simulink model "APFC_FullModel_v22_NoALPF"  (R2025b)
settings: Solver=ode23t  StartTime=0.0  StopTime=50  MaxStep=2e-4  RelTol=1e-3
undefined symbols (not defined in the file): a_dq, ALPF_fs, b_dq, C_B1, C_B2, C_B3, DiscIntNeverNeededParam, dspblkCoreblockFVToolHelper, FLC_deadband_kVAR, gcbh, L_B1, L_B2, L_B3, omega, p, Q_reactor, Rc, tau_Qload, X1
libraries: ee_lib x63, fl_lib x59, nesl_utility x43, dspswit3 x9, eeTransforms x2, fuzblock x1, eeSinusoidalMeasurementV2 x1
(part 1 of 4)
settings Model: Creator=User  LastModifiedBy=User
settings SolverCC: MaxConsecutiveMinStep=1000

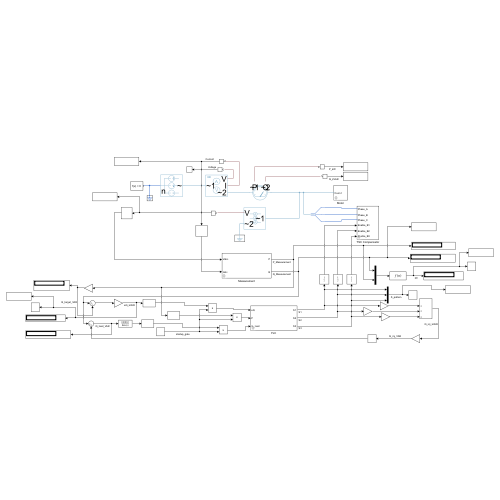
[thumbnail: Simulink's stored preview of the top-level diagram]
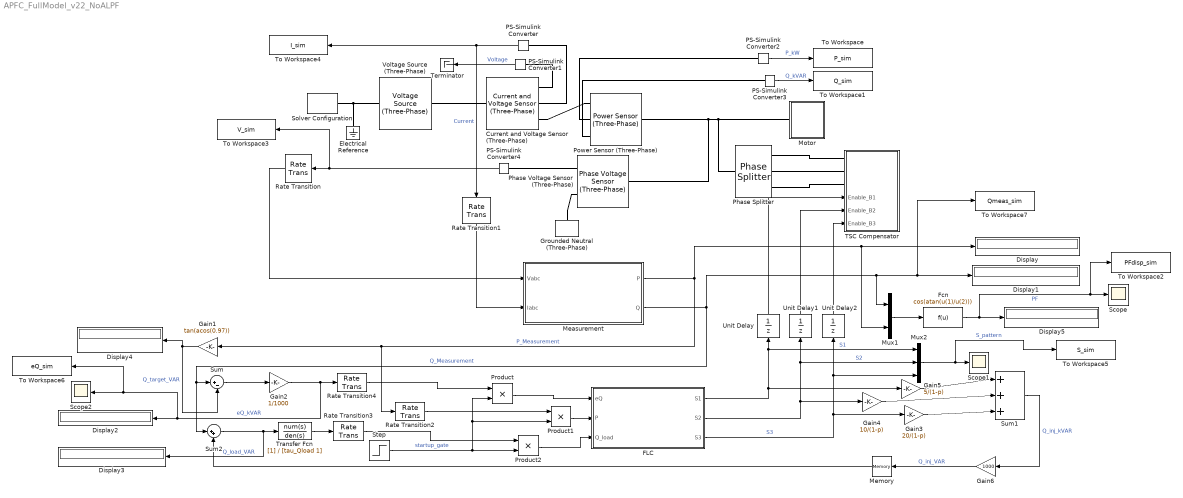
== system APFC_FullModel_v22_NoALPF ==
  Current and Voltage Sensor (Three-Phase) : ee_lib/Sensors & Transducers/Current and Voltage Sensor (Three-Phase)  vMeasurementType=ee.enum.vmeasurement.ll  outputUnit=ee.enum.unit.si  SRated=100e6 A*V  VRated=24e3 V  I_specify=off  I_priority=None  I=[0, 0, 0] A  I_nominal_specify=off  I_nominal_value=1  I_nominal_unit=A  V_specify=off  V_priority=None  V=[0, 0, 0] V  V_nominal_specify=off  V_nominal_value=1  V_nominal_unit=V
      settings: InternalSimscapePortConfiguration="{\"Bottom\":[],\"Left\":[{\"id\":\"N1\",\"label\":\"~1\",\"type\":\"foundation.electrical.three_phase\"}],\"Right\":[{\"id\":\"V_output\",\"label\":\"V\",\"type\":\"output\"},{\"id\":\"I_output\",\"label\":\"I\",\"type\":\"output\"},{\"id\":\"N2\",\"label\":\"~2\",\"type\":\"foundation.electrical.three_phase\"}],\"Top\":[]}"
  Display{,1..5} (6 alike) : Display
  Electrical Reference : fl_lib/Electrical/Electrical Elements/Electrical Reference
  FLC : Subsystem  mask(Fuzzy Logic Controller){}
      mask help: Reads eQ, P, Q_load; fuzzy inference plus deterministic PF-floor; outputs bank commands S1/S2/S3. Parameters sourced from APFC_Parameters.m.
  Fcn : Fcn  Expr=cos(atan(u(1)/u(2)))
  Gain1 : Gain  Gain=tan(acos(0.97))
  Gain2 : Gain  Gain=1/1000
  Gain3 : Gain  Gain=20/(1-p)
  Gain4 : Gain  Gain=10/(1-p)
  Gain5 : Gain  Gain=5/(1-p)
  Gain6 : Gain  Gain=1000
  Grounded Neutral (Three-Phase) : ee_lib/Connectors & References/Grounded Neutral (Three-Phase)
  Measurement : Subsystem  mask(Measurement){}
      mask help: Vabc, Iabc → P, Q. Native Sinusoidal Measurement (PLL, Three-Phase) + Park Transform; alignment-agnostic instantaneous-power computation. Shared PLL angle for both transforms.
  Memory : Memory
  Motor : Subsystem  mask(APFC Motor){n_rpm=1485}
      mask prompts: n_rpm "Rotor speed (rpm)"
      mask help: 30 kW squirrel-cage induction machine with core-loss shunt (Rc), grounded neutral, and speed-imposed mechanical drive. Electrical parameters from APFC_Parameters.m. Rotor speed set via n_rpm.
  Mux1 : Mux  Inputs=2
  Mux2 : Mux  Inputs=3
  PS-Simulink Converter{,1..4} (5 alike) : nesl_utility/PS-Simulink Converter  PhysicalDomain=network_engine_domain  SubClassName=ps_output  LeftPortType=input  RightPortType=output  PseudoPeriodic=off  Frequencies=[]  VectorFormat=inherit  Unit=inherit  AffineConversion=off
  Phase Splitter : ee_lib/Connectors & References/Phase Splitter
  Phase Voltage Sensor (Three-Phase) : ee_lib/Sensors & Transducers/Phase Voltage Sensor (Three-Phase)
  Power Sensor (Three-Phase) : ee_lib/Sensors & Transducers/Power Sensor (Three-Phase)  load_type=ee.enum.passive.type_balanced.balanced  f0=50 Hz
      settings: InternalSimscapePortConfiguration="{\"Bottom\":[],\"Left\":[{\"id\":\"N1\",\"label\":\"~1\",\"type\":\"foundation.electrical.three_phase\"}],\"Right\":[{\"id\":\"N2\",\"label\":\"~2\",\"type\":\"foundation.electrical.three_phase\"}],\"Top\":[{\"id\":\"Pm\",\"label\":\"P\",\"type\":\"output\"},{\"id\":\"Qm\",\"label\":\"Q\",\"type\":\"output\"}]}"
  Product : Product
  Product1 : Product
  Product2 : Product
  Rate Transition : RateTransition  Deterministic=off  OutPortSampleTime=1/12500
  Rate Transition1 : RateTransition  Deterministic=off  OutPortSampleTime=1/12500
  Rate Transition2 : RateTransition  OutPortSampleTime=0.5
  Rate Transition3 : RateTransition  OutPortSampleTime=0.5
  Rate Transition4 : RateTransition  OutPortSampleTime=0.5
  Scope : Scope
      settings: ActiveDisplayYMinimum=-0.12495061956957584  ActiveDisplayYMaximum=1.1249945132855084
  Scope1 : Scope
      settings: ActiveDisplayYMinimum=-0.12499999999999997  ActiveDisplayYMaximum=1.125  DataLoggingVariableName=ScopeData3
  Scope2 : Scope
      settings: ActiveDisplayYMinimum=-28.043898600792488  ActiveDisplayYMaximum=214.93630943141093  DataLoggingVariableName=ScopeData4
  Solver Configuration : nesl_utility/Solver Configuration  PhysicalDomain=network_engine_domain  SubClassName=solver  LeftPortType=input  RightPortType=generic  Tones=[]  Harmonics=[]  SimulateNoise=off  Profile=off  UseLocalSampling=off  EnableSwitchedLinearOptims=on  FrequencyDomain=off  UseCCode=off  RelTol=0.001  AbsTol=0.001  MinStep=1e-09  ToWorkspace=off  RevertToSquareIcSolve=off  NumHomotopyIterations=100  PhasorMode=off  PhasorModeNumHarmonics=1  ConsistencySolver=NEWTON_XTOL_AFTER_FTOL  IndexReductionMethod=DerivativeReplacement  DoDC=off  ResidualTolerance=1e-09  ConsistencyTolSource=GLOBAL  ConsistencyAbsTol=0.001  ConsistencyRelTol=0.001  ConsistencyTolFactor=0.01  UseLocalSolver=off  LocalSolverChoice=NE_BACKWARD_EULER_ADVANCER  ResolveIndetEquations=on  FunctionEvalNumThread=1  LocalSolverSampleTime=0.001  DoFixedCost=off  MaxNonlinIter=3  MaxModeIter=2  ComputeImpulses=off  ImpulseIterations=2  LinearAlgebra=auto  LinearAlgebraNumThread=0  EquationFormulation=NE_TIME_EF  DelaysMemoryBudget=1024  AutomaticFiltering=on  FilteringTimeConstant=0.001  PartitionStorageMethod=AS_NEEDED  PartitionMemoryBudget=1024  PartitionMethod=ROBUST  MultibodyUseLocalSolver=off  MultibodyLocalSolverChoice=ODE1  MultibodyLocalSolverSampleTime=0.001
  Step : Step  Time=25  SampleTime=0.5
  Sum : Sum  Inputs=|+-
  Sum1 : Sum  Inputs=|+++
  Sum2 : Sum  Inputs=|++
  TSC Compensator : Subsystem  mask(TSC Compensator){}
      mask help: Three-phase, delta-connected thyristor-switched capacitor compensator. Three binary-weighted banks: Bank_1 = 5 kVAR, Bank_2 = 10 kVAR, Bank_3 = 20 kVAR (nominal capacitor rating) at 415 V / 50 Hz, 6 % detuned, delivering 5.32 / 10.64 / 21.28 kVAR to the network. Each bank is enabled via Enable_B1/B2/B3 with ZCD-latched transient-free switching. Capacitance and inductance are set inside each bank's Delta_Limb masks — not at this level. Ports: physical Phase_A/B/C; signal Enable_B1/B2/B3.
      settings: PortSchema="{\"entries\":[{\"content\":{\"sides\":[{\"content\":{\"connectorIds\":[\"LConn1\",\"LConn2\",\"LConn3\",\"In1\",\"In2\",\"In3\"]},\"type\":\"ConnectorPlacement.EquallySpacedRectSide\",\"uuid\":\"f449d328-b061-4fce-b527-12937b4bf208\"},{\"content\":{\"side\":\"RIGHT\"},\"type\":\"ConnectorPlacement.EquallySpacedRectSide\",\"uuid\":\"515dffab-51bf-4c86-87e0-d575b9a1f73c\"},{\"content\":{\"side\":\"TOP\"},\"type\":\"ConnectorPlacement.EquallySpacedRectSide\",\"uuid\":\"b4eb947e-b77f-4dcc-ae55-0412ff2259e4\"}]},\"type\":\"ConnectorPlacement.EquallySpacedConnector\",\"uuid\":\"1bf47cce-5631-4349-8217-69cf3260ee1b\"}],\"packageUris\":[\"http://schema.mathworks.com/mf0/Connector/R2020b\"],\"version\":\"1.0\"}"
  Terminator : Terminator
  To Workspace : ToWorkspace  VariableName=P_sim  SampleTime=-1
  To Workspace1 : ToWorkspace  VariableName=Q_sim  SampleTime=-1
  To Workspace2 : ToWorkspace  VariableName=PFdisp_sim  SaveFormat=Timeseries  SampleTime=-1
  To Workspace3 : ToWorkspace  VariableName=V_sim  SampleTime=-1
  To Workspace4 : ToWorkspace  VariableName=I_sim  SampleTime=-1
  To Workspace5 : ToWorkspace  VariableName=S_sim  SaveFormat=Timeseries  SampleTime=-1
  To Workspace6 : ToWorkspace  VariableName=eQ_sim  SaveFormat=Timeseries  SampleTime=-1
  To Workspace7 : ToWorkspace  VariableName=Qmeas_sim  SaveFormat=Timeseries  SampleTime=-1
  Transfer Fcn : TransferFcn  Denominator=[tau_Qload 1]
  Unit Delay : UnitDelay  SampleTime=0.5  HasFrameUpgradeWarning=on
  Unit Delay1 : UnitDelay  SampleTime=0.5  HasFrameUpgradeWarning=on
  Unit Delay2 : UnitDelay  SampleTime=0.5  HasFrameUpgradeWarning=on
  Voltage Source (Three-Phase) : ee_lib/Sources/Voltage Source (Three-Phase)  vline_rms=415 V  shift=0 deg  freq=50 Hz  impedance_option=2  SShortCircuit=1e6 A*V  XR=15  R=0.001 Ohm  L=3.97e-4 H  harmonic_option=1  harmonic_orders=H_orders  harmonic_ratios=H_ratios  G_parasitic=0 1/Ohm  I_specify=off  I_priority=None  I=[0, 0, 0] A  I_nominal_specify=off  I_nominal_value=1  I_nominal_unit=A
  wires:
  PS-Simulink Converter/1 -> To Workspace4/1, Rate Transition1/1  "Current"
  PS-Simulink Converter3/1 -> To Workspace1/1  "Q_kVAR"
  PS-Simulink Converter2/1 -> To Workspace/1  "P_kW"
  PS-Simulink Converter4/1 -> To Workspace3/1, Rate Transition/1
  Rate Transition/1 -> Measurement/1(Vabc)
  Rate Transition1/1 -> Measurement/2(Iabc)
  Measurement/2(Q) -> Sum2/1, Sum/1, Mux1/1, To Workspace7/1, Display1/1  "Q_Measurement"
  Measurement/1(P) -> Rate Transition2/1, Gain1/1, Mux1/2, Display/1  "P_Measurement"
  Gain1/1 -> Sum/2, Display4/1  "Q_target_VAR"
  Sum/1 -> Gain2/1
  Sum1/1 -> Gain6/1  "Q_inj_kVAR"
  Gain6/1 -> Memory/1  "Q_inj_VAR"
  Memory/1 -> Sum2/2
  Gain2/1 -> To Workspace6/1, Scope2/1, Display2/1, Rate Transition4/1  "eQ_kVAR"
  Sum2/1 -> Display3/1, Transfer Fcn/1  "Q_load_VAR"
  Product/1 -> FLC/1(eQ)
  Product1/1 -> FLC/2(P)
  Product2/1 -> FLC/3(Q_load)
  Step/1 -> Product1/2, Product/2, Product2/2  "startup_gate"
  Rate Transition3/1 -> Product2/1
  Rate Transition2/1 -> Product1/1
  Rate Transition4/1 -> Product/1
  FLC/3(S3) -> Unit Delay2/1, Mux2/3, Gain3/1  "S3"
  FLC/2(S2) -> Unit Delay1/1, Mux2/2, Gain4/1  "S2"
  FLC/1(S1) -> Unit Delay/1, Mux2/1, Gain5/1  "S1"
  Gain3/1 -> Sum1/3
  Gain4/1 -> Sum1/2
  Gain5/1 -> Sum1/1
  Unit Delay2/1 -> TSC Compensator/3(Enable_B3)
  Unit Delay1/1 -> TSC Compensator/2(Enable_B2)
  Unit Delay/1 -> TSC Compensator/1(Enable_B1)
  Mux1/1 -> Fcn/1
  Fcn/1 -> To Workspace2/1, Scope/1, Display5/1  "PF"
  Mux2/1 -> To Workspace5/1, Scope1/1  "S_pattern"
  Transfer Fcn/1 -> Rate Transition3/1
  PS-Simulink Converter1/1 -> Terminator/1  "Voltage"
  connections:
  Current and Voltage Sensor (Three-Phase)/RConn3 -- Power Sensor (Three-Phase)/LConn1
  Electrical Reference/LConn1 -- Voltage Source (Three-Phase)/LConn1 -- Solver Configuration/RConn1
  PS-Simulink Converter1/LConn1 -- Current and Voltage Sensor (Three-Phase)/RConn1
  PS-Simulink Converter/LConn1 -- Current and Voltage Sensor (Three-Phase)/RConn2
  Voltage Source (Three-Phase)/RConn1 -- Current and Voltage Sensor (Three-Phase)/LConn1
  Phase Splitter/RConn2 -- TSC Compensator/LConn2
  Phase Splitter/RConn3 -- TSC Compensator/LConn3
  Phase Splitter/RConn1 -- TSC Compensator/LConn1
  Power Sensor (Three-Phase)/RConn1 -- Phase Voltage Sensor (Three-Phase)/LConn1 -- Phase Splitter/LConn1 -- Motor/LConn1
  Grounded Neutral (Three-Phase)/LConn1 -- Phase Voltage Sensor (Three-Phase)/RConn2
  Phase Voltage Sensor (Three-Phase)/RConn1 -- PS-Simulink Converter4/LConn1
  PS-Simulink Converter3/LConn1 -- Power Sensor (Three-Phase)/LConn3
  PS-Simulink Converter2/LConn1 -- Power Sensor (Three-Phase)/LConn2

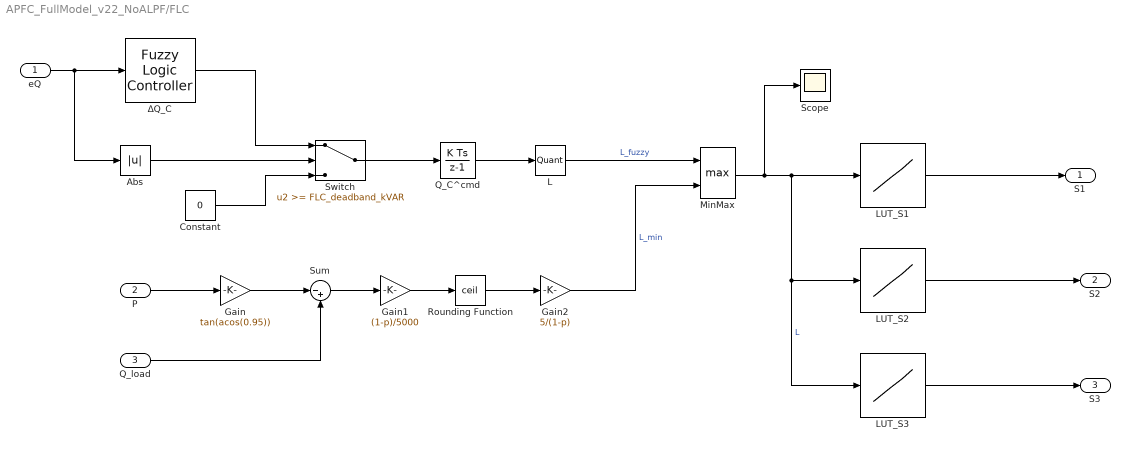
== system APFC_FullModel_v22_NoALPF/FLC ==
  eQ : Inport
  P : Inport  Port=2
  Q_load : Inport  Port=3
  Abs : Abs  SaturateOnIntegerOverflow=off
  Constant : Constant  Value=0
  Gain : Gain  Gain=tan(acos(0.95))
  Gain1 : Gain  Gain=(1-p)/5000
  Gain2 : Gain  Gain=5/(1-p)
  L : Quantizer  QuantizationInterval=5/(1-p)
  LUT_S1 : Lookup_n-D  NumberOfTableDimensions=1  BreakpointsForDimension1=(0:7)*(5/(1-p))  Table=[0 1 0 1 0 1 0 1]  InterpMethod=Flat  InternalRulePriority=Speed  RndMeth=Simplest
  LUT_S2 : Lookup_n-D  NumberOfTableDimensions=1  BreakpointsForDimension1=(0:7)*(5/(1-p))  Table=[0 0 1 1 0 0 1 1]  InterpMethod=Flat  InternalRulePriority=Speed  RndMeth=Simplest
  LUT_S3 : Lookup_n-D  NumberOfTableDimensions=1  BreakpointsForDimension1=(0:7)*(5/(1-p))  Table=[0 0 0 0 1 1 1 1]  InterpMethod=Flat  InternalRulePriority=Speed  RndMeth=Simplest
  MinMax : MinMax  Function=max  Inputs=2
  Q_C^cmd : DiscreteIntegrator  gainval=0.2  SampleTime=0.5  LimitOutput=on  UpperSaturationLimit=35/(1-p)  LowerSaturationLimit=0  ICPrevOutput=DiscIntNeverNeededParam  ICPrevScaledInput=DiscIntNeverNeededParam
  Rounding Function : Rounding  Operator=ceil
  Scope : Scope
      settings: ActiveDisplayYMinimum=5.9574468085106389  ActiveDisplayYMaximum=25.957446808510639  DataLoggingVariableName=ScopeData2
  Sum : Sum  Inputs=|-+
  Switch : Switch  Threshold=FLC_deadband_kVAR  SaturateOnIntegerOverflow=off  InputSameDT=off
  ΔQ_C : fuzblock/Fuzzy Logic  Controller  FIS=fis  OutputSampleNumber=101  DataType=double  UseLookupTable=off  NumBreakpoints=10  FuzzifiedInputs=off  RuleFiringStrengths=off  RuleOutputs=off  AggregatedOutputs=off  SimulateUsing=Interpreted execution  OutOfRangeInputValueMessage=warning  NoRuleFiredMessage=warning  EmptyOutputFuzzySetMessage=warning
  S1 : Outport
  S2 : Outport  Port=2
  S3 : Outport  Port=3
  wires:
  Q_C^cmd/1 -> L/1
  LUT_S3/1 -> S3/1
  eQ/1 -> Abs/1, ΔQ_C/1
  LUT_S1/1 -> S1/1
  LUT_S2/1 -> S2/1
  Switch/1 -> Q_C^cmd/1
  ΔQ_C/1 -> Switch/1
  Abs/1 -> Switch/2
  Constant/1 -> Switch/3
  P/1 -> Gain/1
  Gain/1 -> Sum/1
  Q_load/1 -> Sum/2
  Sum/1 -> Gain1/1
  Gain1/1 -> Rounding Function/1
  Rounding Function/1 -> Gain2/1
  MinMax/1 -> Scope/1, LUT_S3/1, LUT_S2/1, LUT_S1/1  "L"
  L/1 -> MinMax/1  "L_fuzzy"
  Gain2/1 -> MinMax/2  "L_min"

== system APFC_FullModel_v22_NoALPF/Measurement ==
  Vabc : Inport
  Iabc : Inport  Port=2
  Demux : Demux  Outputs=3
  Demux1 : Demux  Outputs=3
  Discrete Transfer Fcn : DiscreteTransferFcn  LoadFcn=dspblkCoreblockFVToolHelper(gcbh,'load');  Numerator=[b_dq]  Denominator=[1 -a_dq]
      settings: CopyFcn=dspblkCoreblockFVToolHelper(gcbh,'copy');  DeleteFcn=dspblkCoreblockFVToolHelper(gcbh,'close');  ModelCloseFcn=dspblkCoreblockFVToolHelper(gcbh,'close');  PreSaveFcn=dspblkCoreblockFVToolHelper(gcbh,'presave');  PostSaveFcn=dspblkCoreblockFVToolHelper(gcbh,'postsave');  CloseFcn=dspblkCoreblockFVToolHelper(gcbh,'close');
  Discrete Transfer Fcn1 : DiscreteTransferFcn  LoadFcn=dspblkCoreblockFVToolHelper(gcbh,'load');  Numerator=[b_dq]  Denominator=[1 -a_dq]
      settings: CopyFcn=dspblkCoreblockFVToolHelper(gcbh,'copy');  DeleteFcn=dspblkCoreblockFVToolHelper(gcbh,'close');  ModelCloseFcn=dspblkCoreblockFVToolHelper(gcbh,'close');  PreSaveFcn=dspblkCoreblockFVToolHelper(gcbh,'presave');  PostSaveFcn=dspblkCoreblockFVToolHelper(gcbh,'postsave');  CloseFcn=dspblkCoreblockFVToolHelper(gcbh,'close');
  Mux2 : Mux
  P-Fcn : Fcn  Expr=1.5*(u(1)*u(3)+u(2)*u(4))
  Park Transform : eeTransforms/Park Transform  AxisAlignment=D-axis  PowerInvariant=off
      settings: LibrarySourceBlock=|
      | ee_sl_lib/Mathematical
      | Transforms/Park Transform
  Park Transform1 : eeTransforms/Park Transform  AxisAlignment=D-axis  PowerInvariant=off
      settings: LibrarySourceBlock=|
      | ee_sl_lib/Mathematical
      | Transforms/Park Transform
  Q-Fcn : Fcn  Expr=1.5*(u(2)*u(3)-u(1)*u(4))
  Scope : Scope
      settings: ActiveDisplayYMinimum=-1  ActiveDisplayYMaximum=1
  "Sinusoidal Measurement (PLL, Three-Phase)" : eeSinusoidalMeasurementV2/Sinusoidal Measurement (PLL, Three-Phase)  InputFilter=on  InputNormalization=off  Kp_LF=1  Ki_LF=10  F0=50  Theta0=0  Ts=1/ALPF_fs
      settings: LibrarySourceBlock=|
      | ee_sl_lib/Measurements/Sinusoidal Measurement
      | (PLL, Three-Phase)
  Terminator{,1..3} (4 alike) : Terminator
  P : Outport
  Q : Outport  Port=2
  wires:
  Park Transform/1 -> Demux/1
  Park Transform1/1 -> Demux1/1
  Demux/1 -> Mux2/1  "Vd"
  P-Fcn/1 -> Discrete Transfer Fcn/1
  Demux/3 -> Terminator2/1
  "Sinusoidal Measurement (PLL, Three-Phase)"/2 -> Scope/1, Park Transform1/2, Park Transform/2
  Demux/2 -> Mux2/2  "Vq"
  "Sinusoidal Measurement (PLL, Three-Phase)"/3 -> Terminator1/1
  Vabc/1 -> Park Transform/1, "Sinusoidal Measurement (PLL, Three-Phase)"/1
  Demux1/3 -> Terminator3/1
  "Sinusoidal Measurement (PLL, Three-Phase)"/1 -> Terminator/1
  Mux2/1 -> Q-Fcn/1, P-Fcn/1
  Iabc/1 -> Park Transform1/1
  Q-Fcn/1 -> Discrete Transfer Fcn1/1
  Discrete Transfer Fcn/1 -> P/1
  Demux1/1 -> Mux2/3  "Id"
  Demux1/2 -> Mux2/4  "Iq"
  Discrete Transfer Fcn1/1 -> Q/1

== system APFC_FullModel_v22_NoALPF/Motor ==
  Grounded Neutral (Three-Phase) : ee_lib/Connectors & References/Grounded Neutral (Three-Phase)
  Ideal Angular Velocity Source : fl_lib/Mechanical/Mechanical Sources/Ideal Angular Velocity Source
  Induction Machine Squirrel Cage : ee_lib/Electromechanical/Asynchronous/Induction Machine Squirrel Cage  port_option=ee.enum.threePhasePort.composite  SRated=SIn_3ph A*V  VRated=415 V  FRated=50 Hz  nPolePairs=2  param_unit=ee.enum.unit.si  squirrel_cage=ee.enum.squirrelcage.Single  zero_sequence=ee.enum.park.zerosequence.exclude  initialization_option=ee.enum.asm.initialization.fluxvariables  Rs=R1 Ohm  Xls=X1 Ohm  pu_Rs=0.0258  pu_Lls=0.0413  Rrd=R2 Ohm  Xlrd=X2 Ohm  pu_Rrd=0.0145  pu_Llrd=0.0424  Rrd1=0.28 Ohm  Xlrd1=0.82 Ohm  Rrd2=0.28 Ohm  Xlrd2=0.82 Ohm  pu_Rrd1=0.0290  pu_Llrd1=0.0848  pu_Rrd2=0.0290  pu_Llrd2=0.0848  Xm=XM Ohm  pu_Lm=1.7562  X0=X1 Ohm  pu_L0=0.0413  saturation_option=ee.enum.saturation.exclude  saturation_i=[0, 4, 9, 18, 25, 34, 50, 68, 95, 120] A  saturation_v=[0, 88, 154, 198, 220, 242, 264, 286, 308, 327] V  pu_saturation_i=[0, .176, .396, .792, 1.1, 1.496, 2.2, 2.992, 4.18, 5.28]  pu_saturation_v=[0, .4, .7, .9, 1, 1.1, 1.2, 1.3, 1.4, 1.4864]  connection_option=ee.enum.Connection.delta  angular_position_specify=off  angular_position_priority=None  angular_position=0 deg  angular_position_nominal_specify=off  angular_position_nominal_value=1  angular_position_nominal_unit=deg  pu_psids_specify=off  pu_psids_priority=None  pu_psids=0  pu_psids_nominal_specify=off  pu_psids_nominal_value=1  pu_psids_nominal_unit=1  pu_psiqs_specify=off  pu_psiqs_priority=None  pu_psiqs=0  pu_psiqs_nominal_specify=off  pu_psiqs_nominal_value=1  pu_psiqs_nominal_unit=1  pu_psi0s_specify=off  pu_psi0s_priority=None  pu_psi0s=0  pu_psi0s_nominal_specify=off  pu_psi0s_nominal_value=1  pu_psi0s_nominal_unit=1  pu_psidr_specify=off  pu_psidr_priority=None  pu_psidr=0  pu_psidr_nominal_specify=off  pu_psidr_nominal_value=1  pu_psidr_nominal_unit=1  pu_psiqr_specify=off  pu_psiqr_priority=None  pu_psiqr=0  pu_psiqr_nominal_specify=off  pu_psiqr_nominal_value=1  pu_psiqr_nominal_unit=1  pu_psidr1_specify=off  pu_psidr1_priority=None  pu_psidr1=0  pu_psidr1_nominal_specify=off  pu_psidr1_nominal_value=1  pu_psidr1_nominal_unit=1  pu_psiqr1_specify=off  pu_psiqr1_priority=None  pu_psiqr1=0  pu_psiqr1_nominal_specify=off  pu_psiqr1_nominal_value=1  pu_psiqr1_nominal_unit=1  pu_psidr2_specify=off  pu_psidr2_priority=None  pu_psidr2=0  pu_psidr2_nominal_specify=off  pu_psidr2_nominal_value=1  pu_psidr2_nominal_unit=1  pu_psiqr2_specify=off  pu_psiqr2_priority=None  pu_psiqr2=0  pu_psiqr2_nominal_specify=off  pu_psiqr2_nominal_value=1  pu_psiqr2_nominal_unit=1  psids_specify=on  psids_priority=Low  psids=0 Wb  psids_nominal_specify=off  psids_nominal_value=1  psids_nominal_unit=Wb  psiqs_specify=on  psiqs_priority=Low  psiqs=0 Wb  psiqs_nominal_specify=off  psiqs_nominal_value=1  psiqs_nominal_unit=Wb  psi0s_specify=off  psi0s_priority=None  psi0s=0 Wb  psi0s_nominal_specify=off  psi0s_nominal_value=1  psi0s_nominal_unit=Wb  psidr_specify=on  psidr_priority=Low  psidr=0 Wb  psidr_nominal_specify=off  psidr_nominal_value=1  psidr_nominal_unit=Wb  psiqr_specify=on  psiqr_priority=Low  psiqr=0 Wb  psiqr_nominal_specify=off  psiqr_nominal_value=1  psiqr_nominal_unit=Wb  psidr1_specify=off  psidr1_priority=None  psidr1=0 Wb  psidr1_nominal_specify=off  psidr1_nominal_value=1  psidr1_nominal_unit=Wb  psiqr1_specify=off  psiqr1_priority=None  psiqr1=0 Wb  psiqr1_nominal_specify=off  psiqr1_nominal_value=1  psiqr1_nominal_unit=Wb  psidr2_specify=off  psidr2_priority=None  psidr2=0 Wb  psidr2_nominal_specify=off  psidr2_nominal_value=1  psidr2_nominal_unit=Wb  psiqr2_specify=off  psiqr2_priority=None  psiqr2=0 Wb  psiqr2_nominal_specify=off  psiqr2_nominal_value=1  psiqr2_nominal_unit=Wb  slip_specify=off  slip_priority=None  slip=0  slip_nominal_specify=off  slip_nominal_value=1  slip_nominal_unit=1  real_power_generated_specify=off  real_power_generated_priority=None  real_power_generated=0 W  real_power_generated_nominal_specify=off  real_power_generated_nominal_value=1  real_power_generated_nominal_unit=W  mechanical_power_consumed_specify=off  mechanical_power_consumed_priority=None  mechanical_power_consumed=0 W  mechanical_power_consumed_nominal_specify=off  mechanical_power_consumed_nominal_value=1  mechanical_power_consumed_nominal_unit=W  Tmeas=298.15 K  alpha=3.93e-3 1/K  alpha_cage=4.4e-3 1/K  stator_thermal_mass=100 J/K  rotor_thermal_mass=200 J/K  temperatureA_specify=off  temperatureA_priority=High  temperatureA=25 degC  temperatureA_nominal_specify=off  temperatureA_nominal_value=1  temperatureA_nominal_unit=degC  temperatureB_specify=off  temperatureB_priority=High  temperatureB=25 degC  temperatureB_nominal_specify=off  temperatureB_nominal_value=1  temperatureB_nominal_unit=degC  temperatureC_specify=off  temperatureC_priority=High  temperatureC=25 degC  temperatureC_nominal_specify=off  temperatureC_nominal_value=1  temperatureC_nominal_unit=degC  temperatureR_specify=off  temperatureR_priority=High  temperatureR=25 degC  temperatureR_nominal_specify=off  temperatureR_nominal_value=1  temperatureR_nominal_unit=degC
      settings: InternalSimscapePortConfiguration="{\"Bottom\":[],\"Left\":[{\"id\":\"R\",\"label\":\"R\",\"type\":\"foundation.mechanical.rotational.rotational\"},{\"id\":\"C\",\"label\":\"C\",\"type\":\"foundation.mechanical.rotational.rotational\"}],\"Right\":[{\"id\":\"pu_output\",\"label\":\"pu\",\"type\":\"output\"},{\"id\":\"N1\",\"label\":\"~1\",\"type\":\"foundation.electrical.three_phase\"},{\"id\":\"N2\",\"label\":\"~2\",\"type\":\"foundation.electrical.three_phase\"}],\"Top\":[]}"
  Inertia : fl_lib/Mechanical/Rotational Elements/Inertia  inertia=J_motor kg*m^2  num_ports=foundation.enum.numPorts2.one  w_specify=off  w_priority=High  w=0 rad/s  w_nominal_specify=off  w_nominal_value=1  w_nominal_unit=rad/s  t_specify=off  t_priority=None  t=0 N*m  t_nominal_specify=off  t_nominal_value=1  t_nominal_unit=N*m
  Mechanical Rotational Reference : fl_lib/Mechanical/Rotational Elements/Mechanical Rotational Reference
  PS Constant : fl_lib/Physical Signals/Sources/PS Constant  constant=(2*pi*n_rpm)/60 rad/s
  PS-Simulink Converter4 : nesl_utility/PS-Simulink Converter  PhysicalDomain=network_engine_domain  SubClassName=ps_output  LeftPortType=input  RightPortType=output  PseudoPeriodic=off  Frequencies=[]  VectorFormat=inherit  Unit=inherit  AffineConversion=off
  Rc : ee_lib/Passive/RLC Assemblies/RLC (Three-Phase)  port_option=ee.enum.threePhasePort.composite  component_structure=ee.enum.rlc.structure.R  R=Rc Ohm  L=1e-3 H  C=1e-6 F  R_parasitic=0 Ohm  G_parasitic=0 1/Ohm  IL_specify=off  IL_priority=High  IL=[0, 0, 0] A  IL_nominal_specify=off  IL_nominal_value=1  IL_nominal_unit=A  VC_specify=off  VC_priority=High  VC=[0, 0, 0] V  VC_nominal_specify=off  VC_nominal_value=1  VC_nominal_unit=V
      settings: InternalSimscapePortConfiguration="{\"Bottom\":[],\"Left\":[{\"id\":\"N1\",\"label\":\"~1\",\"type\":\"foundation.electrical.three_phase\"}],\"Right\":[{\"id\":\"N2\",\"label\":\"~2\",\"type\":\"foundation.electrical.three_phase\"}],\"Top\":[]}"
  Terminator : Terminator
  Conn1 : PMIOPort  Side=Left
  wires:
  PS-Simulink Converter4/1 -> Terminator/1
  connections:
  Inertia/LConn1 -- Ideal Angular Velocity Source/LConn1 -- Induction Machine Squirrel Cage/LConn1
  PS-Simulink Converter4/LConn1 -- Induction Machine Squirrel Cage/RConn1
  Induction Machine Squirrel Cage/RConn2 -- Conn1/RConn1 -- Rc/LConn1
  Mechanical Rotational Reference/LConn1 -- Induction Machine Squirrel Cage/LConn2 -- Ideal Angular Velocity Source/RConn2
  Induction Machine Squirrel Cage/RConn3 -- Rc/RConn1 -- Grounded Neutral (Three-Phase)/LConn1
  Ideal Angular Velocity Source/RConn1 -- PS Constant/RConn1

== system APFC_FullModel_v22_NoALPF/TSC Compensator ==
  Enable_B1 : Inport
  Enable_B2 : Inport  Port=2
  Enable_B3 : Inport  Port=3
  Bank_1 (5 kVAR) : Subsystem
  Bank_2 (10 kVAR) : Subsystem
  Bank_3 (20 kVAR) : Subsystem
  Phase_A : PMIOPort  Side=Left
  Phase_B : PMIOPort  Port=2  Side=Left
  Phase_C : PMIOPort  Port=3  Side=Left
  wires:
  Enable_B3/1 -> Bank_3 (20 kVAR)/1(Enable_B3)
  Enable_B1/1 -> Bank_1 (5 kVAR)/1(Enable_B1)
  Enable_B2/1 -> Bank_2 (10 kVAR)/1(Enable_B2)
  connections:
  Bank_3 (20 kVAR)/LConn2 -- Bank_2 (10 kVAR)/LConn2 -- Bank_1 (5 kVAR)/LConn2 -- Phase_B/RConn1
  Bank_2 (10 kVAR)/LConn1 -- Phase_A/RConn1 -- Bank_1 (5 kVAR)/LConn1 -- Bank_3 (20 kVAR)/LConn1
  Bank_1 (5 kVAR)/LConn3 -- Phase_C/RConn1 -- Bank_2 (10 kVAR)/LConn3 -- Bank_3 (20 kVAR)/LConn3

== system APFC_FullModel_v22_NoALPF/TSC Compensator/Bank_1 (5 kVAR) ==
  Enable_B1 : Inport
  TSC Bank 1 : Subsystem
      mask help:
      | Three-phase delta-connected TSC bank subsystem.
      | Contains three identical Delta_Limb instances (AB, BC, CA) and three line-to-line voltage sensors.
      |
      | Parameters C_val, L_val, and Rd_val are passed to all three Delta_Limb instances.
      | Default values correspond to Bank 1 (5 kVAR) at 415 V / 50 Hz with 6% detuning factor.
      |
      | Electrical ports: Phase_A, Phase_B, Phase_C.
      | Simulink inports: Gate_Drive_AB, Gate_Drive_BC, Gate_Drive_CA.
      | Simulink outports: V_AB, V_BC, V_CA (line voltages),
      | V_C0_AB, V_C0_BC, V_C0_CA (capacitor voltages),
      | V_sw_AB, V_sw_BC, V_sw_CA (thyristor switching voltages) are accessible via internal Scope blocks inside this subsystem.
      |
      | ZCD logic and Enable signals are external to this subsystem.
  ZCD Bank 1 : Subsystem
      mask help:
      | ZCD_Bank subsystem for one three-phase delta-connected TSC bank.
      | Contains ZCD_AB, ZCD_BC, ZCD_CA — one per delta limb.
      |
      | Inports: V_AB, V_BC, V_CA (line voltages from TSC_Bank),
      | V_C0_AB, V_C0_BC, V_C0_CA (capacitor voltages from TSC_Bank),
      | Enable (single switching command, broadcast to all three ZCDs).
      |
      | Outports: Gate_Drive_AB, Gate_Drive_BC, Gate_Drive_CA.
      |
      | One instance required per bank: ZCD_Bank_B1, ZCD_Bank_B2,
      | ZCD_Bank_B3.
  Phase_A : PMIOPort  Side=Left
  Phase_B : PMIOPort  Port=2  Side=Left
  Phase_C : PMIOPort  Port=3  Side=Left
  wires:
  TSC Bank 1/5(V_CA) -> ZCD Bank 1/5(V_CA)  "V_CA_B1"
  TSC Bank 1/2(V_CO_AB) -> ZCD Bank 1/2(V_CO_AB)  "V_CO_AB_B1"
  Enable_B1/1 -> ZCD Bank 1/7(Enable)
  TSC Bank 1/3(V_BC) -> ZCD Bank 1/3(V_BC)  "V_BC_B1"
  TSC Bank 1/1(V_AB) -> ZCD Bank 1/1(V_AB)  "V_AB_B1"
  TSC Bank 1/6(V_CO_CA) -> ZCD Bank 1/6(V_CO_CA)  "V_CO_CA_B1"
  TSC Bank 1/4(V_CO_BC) -> ZCD Bank 1/4(V_CO_BC)  "V_CO_BC_B1"
  ZCD Bank 1/1(Gate_drive_AB) -> TSC Bank 1/1(Gate_Drive_AB)
  ZCD Bank 1/2(Gate_drive_BC) -> TSC Bank 1/2(Gate_Drive_BC)
  ZCD Bank 1/3(Gate_drive_CA) -> TSC Bank 1/3(Gate_Drive_CA)
  connections:
  TSC Bank 1/LConn2 -- Phase_B/RConn1
  TSC Bank 1/LConn3 -- Phase_C/RConn1
  TSC Bank 1/LConn1 -- Phase_A/RConn1

== system APFC_FullModel_v22_NoALPF/TSC Compensator/Bank_2 (10 kVAR) ==
  Enable_B2 : Inport
  TSC Bank 2 : Subsystem
      mask help:
      | Three-phase delta-connected TSC bank subsystem.
      | Contains three identical Delta_Limb instances (AB, BC, CA) and three line-to-line voltage sensors.
      |
      | Parameters C_val, L_val, and Rd_val are passed to all three Delta_Limb instances.
      | Default values correspond to Bank 2 (10 kVAR) at 415 V / 50 Hz with 6% detuning factor.
      |
      | Electrical ports: Phase_A, Phase_B, Phase_C.
      | Simulink inports: Gate_Drive_AB, Gate_Drive_BC, Gate_Drive_CA.
      | Simulink outports: V_AB, V_BC, V_CA (line voltages),
      | V_C0_AB, V_C0_BC, V_C0_CA (capacitor voltages),
      | V_sw_AB, V_sw_BC, V_sw_CA (thyristor switching voltages) are accessible via internal Scope blocks inside this subsystem.
      |
      | ZCD logic and Enable signals are external to this subsystem.
  ZCD Bank 2 : Subsystem
      mask help:
      | ZCD_Bank subsystem for one three-phase delta-connected TSC bank.
      | Contains ZCD_AB, ZCD_BC, ZCD_CA — one per delta limb.
      |
      | Inports: V_AB, V_BC, V_CA (line voltages from TSC_Bank),
      | V_C0_AB, V_C0_BC, V_C0_CA (capacitor voltages from TSC_Bank),
      | Enable (single switching command, broadcast to all three ZCDs).
      |
      | Outports: Gate_Drive_AB, Gate_Drive_BC, Gate_Drive_CA.
      |
      | One instance required per bank: ZCD_Bank_B1, ZCD_Bank_B2,
      | ZCD_Bank_B3.
  Phase_A : PMIOPort  Side=Left
  Phase_B : PMIOPort  Port=2  Side=Left
  Phase_C : PMIOPort  Port=3  Side=Left
  wires:
  TSC Bank 2/2(V_CO_AB) -> ZCD Bank 2/2(V_CO_AB)  "V_CO_AB_B2"
  TSC Bank 2/6(V_CO_CA) -> ZCD Bank 2/6(V_CO_CA)  "V_CO_CA_B2"
  TSC Bank 2/3(V_BC) -> ZCD Bank 2/3(V_BC)  "V_BC_B2"
  TSC Bank 2/5(V_CA) -> ZCD Bank 2/5(V_CA)  "V_CA_B2"
  TSC Bank 2/1(V_AB) -> ZCD Bank 2/1(V_AB)  "V_AB_B2"
  TSC Bank 2/4(V_CO_BC) -> ZCD Bank 2/4(V_CO_BC)  "V_CO_BC_B2"
  Enable_B2/1 -> ZCD Bank 2/7(Enable)
  ZCD Bank 2/1(Gate_drive_AB) -> TSC Bank 2/1(Gate_Drive_AB)
  ZCD Bank 2/2(Gate_drive_BC) -> TSC Bank 2/2(Gate_Drive_BC)
  ZCD Bank 2/3(Gate_drive_CA) -> TSC Bank 2/3(Gate_Drive_CA)
  connections:
  TSC Bank 2/LConn1 -- Phase_A/RConn1
  TSC Bank 2/LConn2 -- Phase_B/RConn1
  TSC Bank 2/LConn3 -- Phase_C/RConn1

== system APFC_FullModel_v22_NoALPF/TSC Compensator/Bank_3 (20 kVAR) ==
  Enable_B3 : Inport
  TSC Bank 3 : Subsystem
      mask help:
      | Three-phase delta-connected TSC bank subsystem.
      | Contains three identical Delta_Limb instances (AB, BC, CA) and three line-to-line voltage sensors.
      |
      | Parameters C_val, L_val, and Rd_val are passed to all three Delta_Limb instances.
      | Default values correspond to Bank 3 (20 kVAR) at 415 V / 50 Hz with 6% detuning factor.
      |
      | Electrical ports: Phase_A, Phase_B, Phase_C.
      | Simulink inports: Gate_Drive_AB, Gate_Drive_BC, Gate_Drive_CA.
      | Simulink outports: V_AB, V_BC, V_CA (line voltages),
      | V_C0_AB, V_C0_BC, V_C0_CA (capacitor voltages),
      | V_sw_AB, V_sw_BC, V_sw_CA (thyristor switching voltages) are accessible via internal Scope blocks inside this subsystem.
      |
      | ZCD logic and Enable signals are external to this subsystem.
  ZCD Bank 3 : Subsystem
      mask help:
      | ZCD_Bank subsystem for one three-phase delta-connected TSC bank.
      | Contains ZCD_AB, ZCD_BC, ZCD_CA — one per delta limb.
      |
      | Inports: V_AB, V_BC, V_CA (line voltages from TSC_Bank),
      | V_C0_AB, V_C0_BC, V_C0_CA (capacitor voltages from TSC_Bank),
      | Enable (single switching command, broadcast to all three ZCDs).
      |
      | Outports: Gate_Drive_AB, Gate_Drive_BC, Gate_Drive_CA.
      |
      | One instance required per bank: ZCD_Bank_B1, ZCD_Bank_B2,
      | ZCD_Bank_B3.
  Phase_A : PMIOPort  Side=Left
  Phase_B : PMIOPort  Port=2  Side=Left
  Phase_C : PMIOPort  Port=3  Side=Left
  wires:
  TSC Bank 3/3(V_BC) -> ZCD Bank 3/3(V_BC)  "V_BC_B3"
  TSC Bank 3/4(V_CO_BC) -> ZCD Bank 3/4(V_CO_BC)  "V_CO_BC_B3"
  TSC Bank 3/6(V_CO_CA) -> ZCD Bank 3/6(V_CO_CA)  "V_CO_CA_B3"
  TSC Bank 3/5(V_CA) -> ZCD Bank 3/5(V_CA)  "V_CA_B3"
  TSC Bank 3/2(V_CO_AB) -> ZCD Bank 3/2(V_CO_AB)  "V_CO_AB_B3"
  TSC Bank 3/1(V_AB) -> ZCD Bank 3/1(V_AB)  "V_AB_B3"
  Enable_B3/1 -> ZCD Bank 3/7(Enable)
  ZCD Bank 3/1(Gate_drive_AB) -> TSC Bank 3/1(Gate_Drive_AB)
  ZCD Bank 3/2(Gate_drive_BC) -> TSC Bank 3/2(Gate_Drive_BC)
  ZCD Bank 3/3(Gate_drive_CA) -> TSC Bank 3/3(Gate_Drive_CA)
  connections:
  Phase_B/RConn1 -- TSC Bank 3/LConn2
  Phase_A/RConn1 -- TSC Bank 3/LConn1
  Phase_C/RConn1 -- TSC Bank 3/LConn3

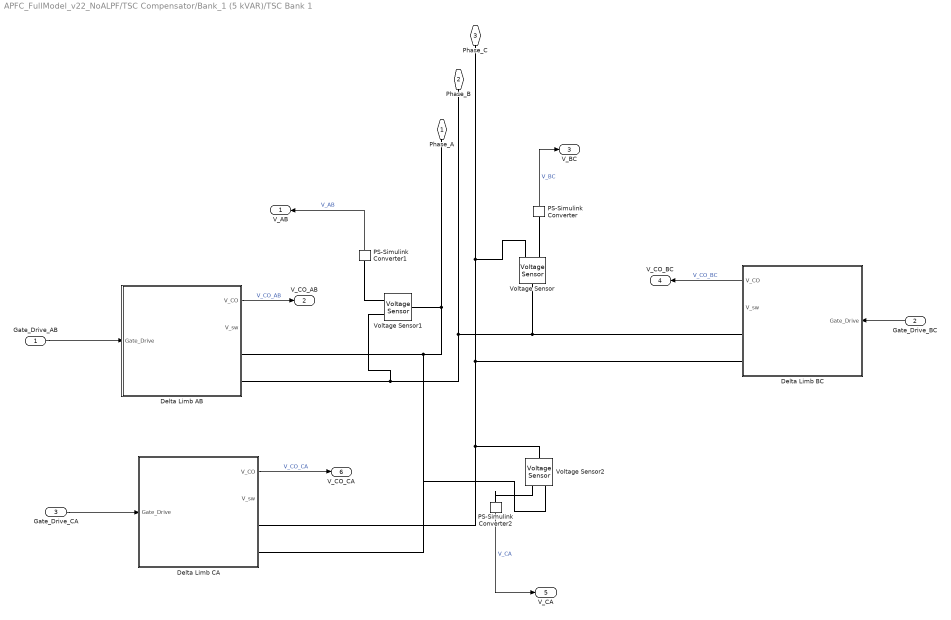
== system APFC_FullModel_v22_NoALPF/TSC Compensator/Bank_1 (5 kVAR)/TSC Bank 1 ==
  Gate_Drive_AB : Inport
  Gate_Drive_BC : Inport  Port=2
  Gate_Drive_CA : Inport  Port=3
  Delta Limb AB : Subsystem  mask{C_val=C_B1, L_val=L_B1, Rd_val=100e3}
      mask prompts: C_val "Capacitance (F)"; L_val "Inductance (H)"; Rd_val "Discharge Resistance (Ohm)"
      mask help:
      | Delta limb of a three-phase delta-connected TSC bank.
      | Contains: anti-parallel thyristor pair, detuning reactor (L_val,
      | R_series = omega*L_val/Q_reactor), shunt capacitor (C_val), parallel discharge
      | resistor (Rd_val), RC snubber (100 Ohm, 0.1 uF).
      |
      | Output signals:
      | V_sw: instantaneous voltage across the anti-parallel thyristor pair.
      | Used as a diagnostic signal to verify transient-free switching.
      | At the moment of firing, V_sw should be at or near zero. After
      | turn-off, V_sw reflects the difference between the line-to-line
      | source voltage and the capacitor voltage V_C0.
      |
      | V_C0: instantaneous voltage across the shunt capacitor. Fed
      | externally to the ZCD comparator as the residual capacitor voltage
      | reference for voltage-matched firing on subsequent switching events.
      |
      | ZCD logic and gate drive signals are external to this subsystem.
      | Default values correspond to Bank 3 (20 kVAR) at 415 V / 50 Hz
      | with 6% detuning factor. Parameter values for Bank 1 (5 kVAR) and
      | Bank 2 (10 kVAR) are assigned by editing the mask dialog at
      | instantiation.
  Delta Limb BC : Subsystem  mask{C_val=C_B1, L_val=L_B1, Rd_val=100e3}
      mask prompts: C_val "Capacitance (F)"; L_val "Inductance (H)"; Rd_val "Discharge Resistance (Ohm)"
      mask help:
      | Delta limb of a three-phase delta-connected TSC bank.
      | Contains: anti-parallel thyristor pair, detuning reactor (L_val,
      | R_series = omega*L_val/Q_reactor), shunt capacitor (C_val), parallel discharge
      | resistor (Rd_val), RC snubber (100 Ohm, 0.1 uF).
      |
      | Output signals:
      | V_sw: instantaneous voltage across the anti-parallel thyristor pair.
      | Used as a diagnostic signal to verify transient-free switching.
      | At the moment of firing, V_sw should be at or near zero. After
      | turn-off, V_sw reflects the difference between the line-to-line
      | source voltage and the capacitor voltage V_C0.
      |
      | V_C0: instantaneous voltage across the shunt capacitor. Fed
      | externally to the ZCD comparator as the residual capacitor voltage
      | reference for voltage-matched firing on subsequent switching events.
      |
      | ZCD logic and gate drive signals are external to this subsystem.
      | Default values correspond to Bank 3 (20 kVAR) at 415 V / 50 Hz
      | with 6% detuning factor. Parameter values for Bank 1 (5 kVAR) and
      | Bank 2 (10 kVAR) are assigned by editing the mask dialog at
      | instantiation.
  Delta Limb CA : Subsystem  mask{C_val=C_B1, L_val=L_B1, Rd_val=100e3}
      mask prompts: C_val "Capacitance (F)"; L_val "Inductance (H)"; Rd_val "Discharge Resistance (Ohm)"
      mask help:
      | Delta limb of a three-phase delta-connected TSC bank.
      | Contains: anti-parallel thyristor pair, detuning reactor (L_val,
      | R_series = omega*L_val/Q_reactor), shunt capacitor (C_val), parallel discharge
      | resistor (Rd_val), RC snubber (100 Ohm, 0.1 uF).
      |
      | Output signals:
      | V_sw: instantaneous voltage across the anti-parallel thyristor pair.
      | Used as a diagnostic signal to verify transient-free switching.
      | At the moment of firing, V_sw should be at or near zero. After
      | turn-off, V_sw reflects the difference between the line-to-line
      | source voltage and the capacitor voltage V_C0.
      |
      | V_C0: instantaneous voltage across the shunt capacitor. Fed
      | externally to the ZCD comparator as the residual capacitor voltage
      | reference for voltage-matched firing on subsequent switching events.
      |
      | ZCD logic and gate drive signals are external to this subsystem.
      | Default values correspond to Bank 3 (20 kVAR) at 415 V / 50 Hz
      | with 6% detuning factor. Parameter values for Bank 1 (5 kVAR) and
      | Bank 2 (10 kVAR) are assigned by editing the mask dialog at
      | instantiation.
  PS-Simulink Converter : nesl_utility/PS-Simulink Converter  PhysicalDomain=network_engine_domain  SubClassName=ps_output  LeftPortType=input  RightPortType=output  PseudoPeriodic=off  Frequencies=[]  VectorFormat=inherit  Unit=inherit  AffineConversion=off
  PS-Simulink Converter1 : nesl_utility/PS-Simulink Converter  PhysicalDomain=network_engine_domain  SubClassName=ps_output  LeftPortType=input  RightPortType=output  PseudoPeriodic=off  Frequencies=[]  VectorFormat=inherit  Unit=inherit  AffineConversion=off
  PS-Simulink Converter2 : nesl_utility/PS-Simulink Converter  PhysicalDomain=network_engine_domain  SubClassName=ps_output  LeftPortType=input  RightPortType=output  PseudoPeriodic=off  Frequencies=[]  VectorFormat=inherit  Unit=inherit  AffineConversion=off
  Voltage Sensor : fl_lib/Electrical/Electrical Sensors/Voltage Sensor
  Voltage Sensor1 : fl_lib/Electrical/Electrical Sensors/Voltage Sensor
  Voltage Sensor2 : fl_lib/Electrical/Electrical Sensors/Voltage Sensor
  Phase_A : PMIOPort  Side=Left
  Phase_B : PMIOPort  Port=2  Side=Left
  Phase_C : PMIOPort  Port=3  Side=Left
  V_AB : Outport
  V_CO_AB : Outport  Port=2
  V_BC : Outport  Port=3
  V_CO_BC : Outport  Port=4
  V_CA : Outport  Port=5
  V_CO_CA : Outport  Port=6
  wires:
  Delta Limb BC/1(V_CO) -> V_CO_BC/1  "V_CO_BC"
  PS-Simulink Converter/1 -> V_BC/1  "V_BC"
  Gate_Drive_CA/1 -> Delta Limb CA/1(Gate_Drive)
  PS-Simulink Converter1/1 -> V_AB/1  "V_AB"
  Delta Limb AB/1(V_CO) -> V_CO_AB/1  "V_CO_AB"
  Delta Limb CA/1(V_CO) -> V_CO_CA/1  "V_CO_CA"
  Gate_Drive_BC/1 -> Delta Limb BC/1(Gate_Drive)
  Gate_Drive_AB/1 -> Delta Limb AB/1(Gate_Drive)
  PS-Simulink Converter2/1 -> V_CA/1  "V_CA"
  connections:
  Delta Limb BC/RConn1 -- Voltage Sensor/LConn1 -- Phase_B/RConn1 -- Voltage Sensor1/RConn2 -- Delta Limb AB/RConn2
  Voltage Sensor1/RConn1 -- PS-Simulink Converter1/LConn1
  PS-Simulink Converter2/LConn1 -- Voltage Sensor2/RConn1
  Voltage Sensor/RConn2 -- Phase_C/RConn1 -- Delta Limb BC/RConn2 -- Voltage Sensor2/LConn1 -- Delta Limb CA/RConn1
  Voltage Sensor/RConn1 -- PS-Simulink Converter/LConn1
  Voltage Sensor1/LConn1 -- Phase_A/RConn1 -- Voltage Sensor2/RConn2 -- Delta Limb CA/RConn2 -- Delta Limb AB/RConn1

== system APFC_FullModel_v22_NoALPF/TSC Compensator/Bank_1 (5 kVAR)/ZCD Bank 1 ==
  V_AB : Inport
  V_CO_AB : Inport  Port=2
  V_BC : Inport  Port=3
  V_CO_BC : Inport  Port=4
  V_CA : Inport  Port=5
  V_CO_CA : Inport  Port=6
  Enable : Inport  Port=7
  ZCD AB : Subsystem
      mask help:
      | Zero-Crossing Detection (ZCD) subsystem for one delta limb of a
      | three-phase delta-connected TSC bank.
      |
      | Implements voltage-matched firing logic for transient-free
      | thyristor switching.
      |
      | Inputs:
      | V_source: instantaneous line-to-line voltage for this limb,
      | fed through a Unit Delay (T_s = 0.0001 s) to the comparator.
      |
      | V_C0: residual capacitor voltage from the corresponding
      | Delta_Limb instance, fed through a Unit Delay (T_s = 0.0001 s)
      | to the comparator.
      |
      | Enable: FLC switching command (S = 1 to arm, S = 0 to inhibit).
      | Set to Constant = 1 for open-loop testing.
      |
      | Output:
      | Gate_drive: firing pulse issued when V_source >= V_C0 on a
      | rising edge, AND Enable = 1. Fed to the Gate_drive inport of
      | the corresponding Delta_Limb instance.
      |
      | Internal blocks: Unit Delay (x2), Relational Operator (>=),
      | Zero-Order Hold (T_s = 0.0001 s), Edge Detector (rising edge),
      | AND gate.
      |
      | One instance required per delta limb: ZCD_AB, ZCD_BC, ZCD_CA.
  ZCD BC : Subsystem
      mask help:
      | Zero-Crossing Detection (ZCD) subsystem for one delta limb of a
      | three-phase delta-connected TSC bank.
      |
      | Implements voltage-matched firing logic for transient-free
      | thyristor switching.
      |
      | Inputs:
      | V_source: instantaneous line-to-line voltage for this limb,
      | fed through a Unit Delay (T_s = 0.0001 s) to the comparator.
      |
      | V_C0: residual capacitor voltage from the corresponding
      | Delta_Limb instance, fed through a Unit Delay (T_s = 0.0001 s)
      | to the comparator.
      |
      | Enable: FLC switching command (S = 1 to arm, S = 0 to inhibit).
      | Set to Constant = 1 for open-loop testing.
      |
      | Output:
      | Gate_drive: firing pulse issued when V_source >= V_C0 on a
      | rising edge, AND Enable = 1. Fed to the Gate_drive inport of
      | the corresponding Delta_Limb instance.
      |
      | Internal blocks: Unit Delay (x2), Relational Operator (>=),
      | Zero-Order Hold (T_s = 0.0001 s), Edge Detector (rising edge),
      | AND gate.
      |
      | One instance required per delta limb: ZCD_AB, ZCD_BC, ZCD_CA.
  ZCD CA : Subsystem
      mask help:
      | Zero-Crossing Detection (ZCD) subsystem for one delta limb of a
      | three-phase delta-connected TSC bank.
      |
      | Implements voltage-matched firing logic for transient-free
      | thyristor switching.
      |
      | Inputs:
      | V_source: instantaneous line-to-line voltage for this limb,
      | fed through a Unit Delay (T_s = 0.0001 s) to the comparator.
      |
      | V_C0: residual capacitor voltage from the corresponding
      | Delta_Limb instance, fed through a Unit Delay (T_s = 0.0001 s)
      | to the comparator.
      |
      | Enable: FLC switching command (S = 1 to arm, S = 0 to inhibit).
      | Set to Constant = 1 for open-loop testing.
      |
      | Output:
      | Gate_drive: firing pulse issued when V_source >= V_C0 on a
      | rising edge, AND Enable = 1. Fed to the Gate_drive inport of
      | the corresponding Delta_Limb instance.
      |
      | Internal blocks: Unit Delay (x2), Relational Operator (>=),
      | Zero-Order Hold (T_s = 0.0001 s), Edge Detector (rising edge),
      | AND gate.
      |
      | One instance required per delta limb: ZCD_AB, ZCD_BC, ZCD_CA.
  Gate_drive_AB : Outport
  Gate_drive_BC : Outport  Port=2
  Gate_drive_CA : Outport  Port=3
  wires:
  V_BC/1 -> ZCD BC/2(V_BC)
  Enable/1 -> ZCD AB/3(Enable), ZCD CA/3(Enable), ZCD BC/3(Enable)
  V_CO_BC/1 -> ZCD BC/1(V_CO_BC)
  V_CA/1 -> ZCD CA/2(V_CA)
  V_AB/1 -> ZCD AB/2(V_AB)
  ZCD BC/1(Gate_drive_BC) -> Gate_drive_BC/1
  V_CO_CA/1 -> ZCD CA/1(V_CO_CA)
  ZCD AB/1(Gate_drive_AB) -> Gate_drive_AB/1
  V_CO_AB/1 -> ZCD AB/1(V_CO_AB)
  ZCD CA/1(Gate_drive_CA) -> Gate_drive_CA/1

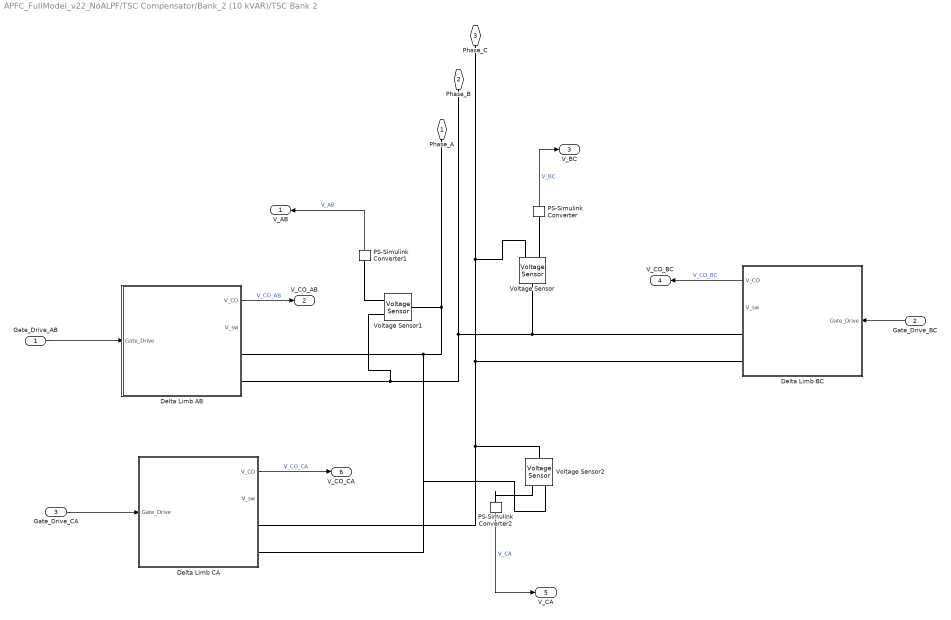
== system APFC_FullModel_v22_NoALPF/TSC Compensator/Bank_2 (10 kVAR)/TSC Bank 2 ==
  Gate_Drive_AB : Inport
  Gate_Drive_BC : Inport  Port=2
  Gate_Drive_CA : Inport  Port=3
  Delta Limb AB : Subsystem  mask{C_val=C_B2, L_val=L_B2, Rd_val=100e3}
      mask prompts: C_val "Capacitance (F)"; L_val "Inductance (H)"; Rd_val "Discharge Resistance (Ohm)"
      mask help:
      | Delta limb of a three-phase delta-connected TSC bank.
      | Contains: anti-parallel thyristor pair, detuning reactor (L_val,
      | R_series = omega*L_val/Q_reactor), shunt capacitor (C_val), parallel discharge
      | resistor (Rd_val), RC snubber (100 Ohm, 0.1 uF).
      |
      | Output signals:
      | V_sw: instantaneous voltage across the anti-parallel thyristor pair.
      | Used as a diagnostic signal to verify transient-free switching.
      | At the moment of firing, V_sw should be at or near zero. After
      | turn-off, V_sw reflects the difference between the line-to-line
      | source voltage and the capacitor voltage V_C0.
      |
      | V_C0: instantaneous voltage across the shunt capacitor. Fed
      | externally to the ZCD comparator as the residual capacitor voltage
      | reference for voltage-matched firing on subsequent switching events.
      |
      | ZCD logic and gate drive signals are external to this subsystem.
      | Default values correspond to Bank 3 (20 kVAR) at 415 V / 50 Hz
      | with 6% detuning factor. Parameter values for Bank 1 (5 kVAR) and
      | Bank 2 (10 kVAR) are assigned by editing the mask dialog at
      | instantiation.
  Delta Limb BC : Subsystem  mask{C_val=C_B2, L_val=L_B2, Rd_val=100e3}
      mask prompts: C_val "Capacitance (F)"; L_val "Inductance (H)"; Rd_val "Discharge Resistance (Ohm)"
      mask help:
      | Delta limb of a three-phase delta-connected TSC bank.
      | Contains: anti-parallel thyristor pair, detuning reactor (L_val,
      | R_series = omega*L_val/Q_reactor), shunt capacitor (C_val), parallel discharge
      | resistor (Rd_val), RC snubber (100 Ohm, 0.1 uF).
      |
      | Output signals:
      | V_sw: instantaneous voltage across the anti-parallel thyristor pair.
      | Used as a diagnostic signal to verify transient-free switching.
      | At the moment of firing, V_sw should be at or near zero. After
      | turn-off, V_sw reflects the difference between the line-to-line
      | source voltage and the capacitor voltage V_C0.
      |
      | V_C0: instantaneous voltage across the shunt capacitor. Fed
      | externally to the ZCD comparator as the residual capacitor voltage
      | reference for voltage-matched firing on subsequent switching events.
      |
      | ZCD logic and gate drive signals are external to this subsystem.
      | Default values correspond to Bank 3 (20 kVAR) at 415 V / 50 Hz
      | with 6% detuning factor. Parameter values for Bank 1 (5 kVAR) and
      | Bank 2 (10 kVAR) are assigned by editing the mask dialog at
      | instantiation.
  Delta Limb CA : Subsystem  mask{C_val=C_B2, L_val=L_B2, Rd_val=100e3}
      mask prompts: C_val "Capacitance (F)"; L_val "Inductance (H)"; Rd_val "Discharge Resistance (Ohm)"
      mask help:
      | Delta limb of a three-phase delta-connected TSC bank.
      | Contains: anti-parallel thyristor pair, detuning reactor (L_val,
      | R_series = omega*L_val/Q_reactor), shunt capacitor (C_val), parallel discharge
      | resistor (Rd_val), RC snubber (100 Ohm, 0.1 uF).
      |
      | Output signals:
      | V_sw: instantaneous voltage across the anti-parallel thyristor pair.
      | Used as a diagnostic signal to verify transient-free switching.
      | At the moment of firing, V_sw should be at or near zero. After
      | turn-off, V_sw reflects the difference between the line-to-line
      | source voltage and the capacitor voltage V_C0.
      |
      | V_C0: instantaneous voltage across the shunt capacitor. Fed
      | externally to the ZCD comparator as the residual capacitor voltage
      | reference for voltage-matched firing on subsequent switching events.
      |
      | ZCD logic and gate drive signals are external to this subsystem.
      | Default values correspond to Bank 3 (20 kVAR) at 415 V / 50 Hz
      | with 6% detuning factor. Parameter values for Bank 1 (5 kVAR) and
      | Bank 2 (10 kVAR) are assigned by editing the mask dialog at
      | instantiation.
  PS-Simulink Converter : nesl_utility/PS-Simulink Converter  PhysicalDomain=network_engine_domain  SubClassName=ps_output  LeftPortType=input  RightPortType=output  PseudoPeriodic=off  Frequencies=[]  VectorFormat=inherit  Unit=inherit  AffineConversion=off
  PS-Simulink Converter1 : nesl_utility/PS-Simulink Converter  PhysicalDomain=network_engine_domain  SubClassName=ps_output  LeftPortType=input  RightPortType=output  PseudoPeriodic=off  Frequencies=[]  VectorFormat=inherit  Unit=inherit  AffineConversion=off
  PS-Simulink Converter2 : nesl_utility/PS-Simulink Converter  PhysicalDomain=network_engine_domain  SubClassName=ps_output  LeftPortType=input  RightPortType=output  PseudoPeriodic=off  Frequencies=[]  VectorFormat=inherit  Unit=inherit  AffineConversion=off
  Voltage Sensor : fl_lib/Electrical/Electrical Sensors/Voltage Sensor
  Voltage Sensor1 : fl_lib/Electrical/Electrical Sensors/Voltage Sensor
  Voltage Sensor2 : fl_lib/Electrical/Electrical Sensors/Voltage Sensor
  Phase_A : PMIOPort  Side=Left
  Phase_B : PMIOPort  Port=2  Side=Left
  Phase_C : PMIOPort  Port=3  Side=Left
  V_AB : Outport
  V_CO_AB : Outport  Port=2
  V_BC : Outport  Port=3
  V_CO_BC : Outport  Port=4
  V_CA : Outport  Port=5
  V_CO_CA : Outport  Port=6
  wires:
  Delta Limb BC/1(V_CO) -> V_CO_BC/1  "V_CO_BC"
  PS-Simulink Converter/1 -> V_BC/1  "V_BC"
  Gate_Drive_CA/1 -> Delta Limb CA/1(Gate_Drive)
  PS-Simulink Converter1/1 -> V_AB/1  "V_AB"
  Delta Limb AB/1(V_CO) -> V_CO_AB/1  "V_CO_AB"
  Delta Limb CA/1(V_CO) -> V_CO_CA/1  "V_CO_CA"
  Gate_Drive_BC/1 -> Delta Limb BC/1(Gate_Drive)
  Gate_Drive_AB/1 -> Delta Limb AB/1(Gate_Drive)
  PS-Simulink Converter2/1 -> V_CA/1  "V_CA"
  connections:
  Delta Limb BC/RConn1 -- Voltage Sensor/LConn1 -- Phase_B/RConn1 -- Voltage Sensor1/RConn2 -- Delta Limb AB/RConn2
  Voltage Sensor1/RConn1 -- PS-Simulink Converter1/LConn1
  PS-Simulink Converter2/LConn1 -- Voltage Sensor2/RConn1
  Voltage Sensor/RConn2 -- Phase_C/RConn1 -- Delta Limb BC/RConn2 -- Voltage Sensor2/LConn1 -- Delta Limb CA/RConn1
  Voltage Sensor/RConn1 -- PS-Simulink Converter/LConn1
  Voltage Sensor1/LConn1 -- Phase_A/RConn1 -- Voltage Sensor2/RConn2 -- Delta Limb CA/RConn2 -- Delta Limb AB/RConn1
